simulink model "Basic_Simulink_Hinf_model"  (R2019a)
settings: Solver=VariableStepAuto  StartTime=0.0  StopTime=100  RelTol=1e-3
undefined symbols (not defined in the file or in its folder): commandError, disterbance, Gc, MeasurementNoise, plant
settings Model: SimulationMode=accelerator  Creator=martin  LastModifiedBy=martin

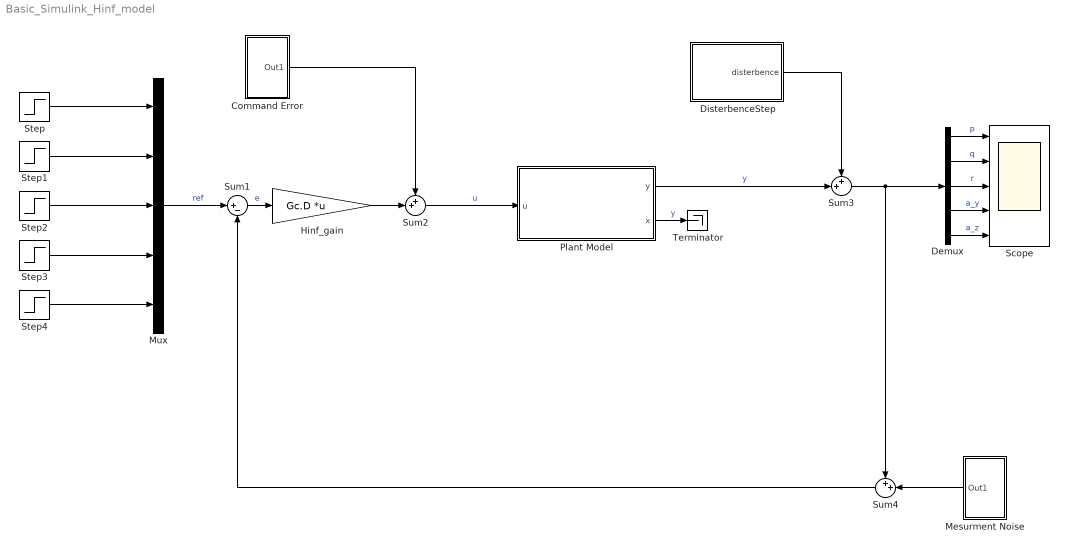
== system Basic_Simulink_Hinf_model ==
  Command Error : Subsystem
  Demux : Demux  Outputs=5
  DisterbenceStep : Subsystem  Variant=on  VariantControl=Variant1
  Hinf_gain : Gain  Gain=Gc.D  Multiplication=Matrix(K*u) (u vector)
  Mesurment Noise : Subsystem
  Mux : Mux  Inputs=5
  Plant Model : Subsystem  mask{plant=plant, IC=[0,0,0,0,0]'}
      mask prompts: plant "Plant SS Object"; IC "Inital Conditions"
  Scope : Scope  NumInputPorts=5
  Step : Step  Time=15  SampleTime=0
  Step1 : Step  Time=25  SampleTime=0
  Step2 : Step  Time=35  SampleTime=0
  Step3 : Step  Time=45  SampleTime=0
  Step4 : Step  Time=55  SampleTime=0
  Sum1 : Sum  Inputs=|+-
  Sum2 : Sum  Inputs=++|
  Sum3 : Sum  Inputs=++|
  Sum4 : Sum  Inputs=++|
  Terminator : Terminator
  wires:
  Sum2/1 -> Plant Model/1(u)  "u"
  Plant Model/2(x) -> Terminator/1  "y"
  Step/1 -> Mux/1
  Plant Model/1(y) -> Sum3/2  "y"
  Mux/1 -> Sum1/1  "ref"
  Step1/1 -> Mux/2
  Step2/1 -> Mux/3
  Sum3/1 -> Sum4/1, Demux/1
  Command Error/1(Out1) -> Sum2/1
  Mesurment Noise/1(Out1) -> Sum4/2
  Sum1/1 -> Hinf_gain/1  "e"
  Hinf_gain/1 -> Sum2/2
  Demux/5 -> Scope/5  "a_z"
  Demux/4 -> Scope/4  "a_y"
  Demux/3 -> Scope/3  "r"
  Demux/2 -> Scope/2  "q"
  Demux/1 -> Scope/1  "p"
  DisterbenceStep/1(disterbence) -> Sum3/1
  Step4/1 -> Mux/5
  Step3/1 -> Mux/4
  Sum4/1 -> Sum1/2

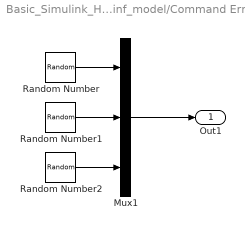
== system Basic_Simulink_Hinf_model/Command Error ==
  Mux1 : Mux  Inputs=3
  Random Number : RandomNumber  Variance=commandError.xi  SampleTime=0.1
  Random Number1 : RandomNumber  Variance=commandError.eta  SampleTime=0.1
  Random Number2 : RandomNumber  Variance=commandError.zeta  SampleTime=0.1
  Out1 : Outport
  wires:
  Random Number/1 -> Mux1/1
  Random Number1/1 -> Mux1/2
  Mux1/1 -> Out1/1
  Random Number2/1 -> Mux1/3

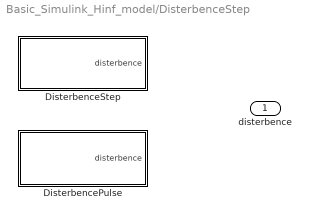
== system Basic_Simulink_Hinf_model/DisterbenceStep ==
  DisterbencePulse : Subsystem  VariantControl=VC_Disterbance_Pulse
  DisterbenceStep : Subsystem  VariantControl=VC_Disterbance_Step
  disterbence : Outport

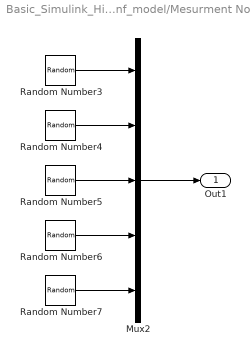
== system Basic_Simulink_Hinf_model/Mesurment Noise ==
  Mux2 : Mux  Inputs=5
  Random Number3 : RandomNumber  Variance=MeasurementNoise.x_p  SampleTime=0.1
  Random Number4 : RandomNumber  Variance=MeasurementNoise.x_q  SampleTime=0.1
  Random Number5 : RandomNumber  Variance=MeasurementNoise.x_r  SampleTime=0.1
  Random Number6 : RandomNumber  Variance=MeasurementNoise.x_w  SampleTime=0.1
  Random Number7 : RandomNumber  Variance=MeasurementNoise.x_v  SampleTime=0.1
  Out1 : Outport
  wires:
  Random Number3/1 -> Mux2/1
  Random Number4/1 -> Mux2/2
  Random Number6/1 -> Mux2/4
  Mux2/1 -> Out1/1
  Random Number7/1 -> Mux2/5
  Random Number5/1 -> Mux2/3

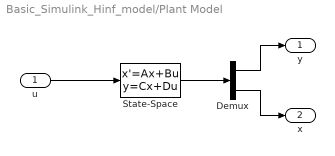
== system Basic_Simulink_Hinf_model/Plant Model ==
  u : Inport
  Demux : Demux  Outputs=[5,5]
  State-Space : StateSpace  A=plant.A  B=plant.B  C=plant.C  D=plant.D  InitialCondition=IC
  y : Outport
  x : Outport  Port=2
  wires:
  State-Space/1 -> Demux/1
  u/1 -> State-Space/1
  Demux/1 -> y/1
  Demux/2 -> x/1

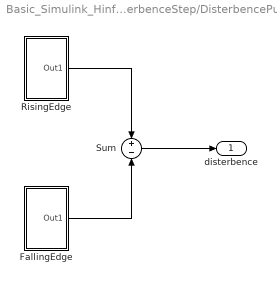
== system Basic_Simulink_Hinf_model/DisterbenceStep/DisterbencePulse ==
  FallingEdge : Subsystem
  RisingEdge : Subsystem
  Sum : Sum  Inputs=+|-
  disterbence : Outport
  wires:
  FallingEdge/1(Out1) -> Sum/2
  RisingEdge/1(Out1) -> Sum/1
  Sum/1 -> disterbence/1

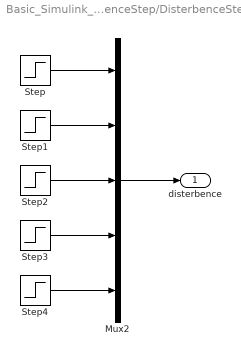
== system Basic_Simulink_Hinf_model/DisterbenceStep/DisterbenceStep ==
  Mux2 : Mux  Inputs=5
  Step : Step  Time=disterbance.time.x_p  After=disterbance.size.x_p  SampleTime=0
  Step1 : Step  Time=disterbance.time.x_q  After=disterbance.size.x_q  SampleTime=0
  Step2 : Step  Time=disterbance.time.x_r  After=disterbance.size.x_r  SampleTime=0
  Step3 : Step  Time=disterbance.time.x_w  After=disterbance.size.x_w  SampleTime=0
  Step4 : Step  Time=disterbance.time.x_v  After=disterbance.size.x_v  SampleTime=0
  disterbence : Outport
  wires:
  Step2/1 -> Mux2/3
  Step4/1 -> Mux2/5
  Mux2/1 -> disterbence/1
  Step3/1 -> Mux2/4
  Step1/1 -> Mux2/2
  Step/1 -> Mux2/1

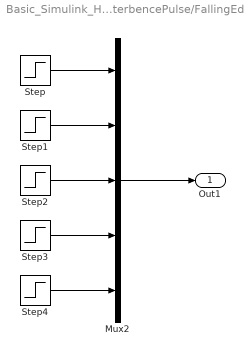
== system Basic_Simulink_Hinf_model/DisterbenceStep/DisterbencePulse/FallingEdge ==
  Mux2 : Mux  Inputs=5
  Step : Step  Time=disterbance.time.x_p + disterbance.duration  After=disterbance.size.x_p  SampleTime=0
  Step1 : Step  Time=disterbance.time.x_q + disterbance.duration  After=disterbance.size.x_q  SampleTime=0
  Step2 : Step  Time=disterbance.time.x_r + disterbance.duration  After=disterbance.size.x_r  SampleTime=0
  Step3 : Step  Time=disterbance.time.x_w + disterbance.duration  After=disterbance.size.x_w  SampleTime=0
  Step4 : Step  Time=disterbance.time.x_v + disterbance.duration  After=disterbance.size.x_v  SampleTime=0
  Out1 : Outport
  wires:
  Step2/1 -> Mux2/3
  Step/1 -> Mux2/1
  Step4/1 -> Mux2/5
  Step3/1 -> Mux2/4
  Step1/1 -> Mux2/2
  Mux2/1 -> Out1/1

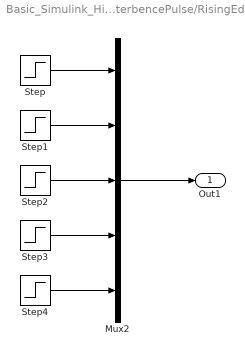
== system Basic_Simulink_Hinf_model/DisterbenceStep/DisterbencePulse/RisingEdge ==
  Mux2 : Mux  Inputs=5
  Step : Step  Time=disterbance.time.x_p  After=disterbance.size.x_p  SampleTime=0
  Step1 : Step  Time=disterbance.time.x_q  After=disterbance.size.x_q  SampleTime=0
  Step2 : Step  Time=disterbance.time.x_r  After=disterbance.size.x_r  SampleTime=0
  Step3 : Step  Time=disterbance.time.x_w  After=disterbance.size.x_w  SampleTime=0
  Step4 : Step  Time=disterbance.time.x_v  After=disterbance.size.x_v  SampleTime=0
  Out1 : Outport
  wires:
  Mux2/1 -> Out1/1
  Step1/1 -> Mux2/2
  Step3/1 -> Mux2/4
  Step4/1 -> Mux2/5
  Step/1 -> Mux2/1
  Step2/1 -> Mux2/3
